simulink model "transfer_function_calculation"  (R2016a)
settings: Solver=VariableStepAuto  StartTime=0.0  StopTime=5  RelTol=1e-3
values from neighbouring files (symbols this model uses):
  a = .7    (= 0.7)    [PM_1_5MW_syn_27.m]
  Flux = 5.8264    [PM_1_5MW_syn_27.m]
  Id_set = 500    [PM_1_5MW_syn_27.m]
  Iq_set = -2200    [PM_1_5MW_syn_27.m]
  L = .0001    (= 0.0001)    [PM_1_5MW_syn_27.m]
  Ld = 0.001575    [PM_1_5MW_syn_27.m]
  Lq = 0.001575    [PM_1_5MW_syn_27.m]
  mn = 60000    [PM_1_5MW_syn_27.m]
  p = 26    [PM_1_5MW_syn_27.m]
  Rs = 0.000821    [PM_1_5MW_syn_27.m]
  Sollkurve_M_Optimum = [0 57121 101549 158670 228485 310994 406196 514092 634681 767965 810425 823386 ... (13 elements, 13x1)]    [Lookup_M_n.mat]
  Sollkurve_nGen_Optimum = [0 5 7 9 11 12 14 16 18 20 20.07 20.2 ... (13 elements, 13x1)]    [Lookup_M_n.mat]
  Speed_set = w_m    (= 2.10172548525)    [PM_1_5MW_syn_27.m]
  Ts_Power = 5.000000000000000e-06    (= 5e-06)    [PM_1_5MW_syn_27.m]
  Vdc = 1200    [PM_1_5MW_syn_27.m]
  Vh = Vm/6*0    (= 0)    [PM_1_5MW_syn_27.m]
undefined symbols (not defined in the file or in its folder): C2, Esw_Erec, Esw_Off, Esw_On, Page_Temp_C
undefined symbols (not defined in the file): Ts_Control, z
libraries: fl_lib x84, powerlib_meascontrol x58, simulink x56, nesl_utility x36, powerlib x33, simulink_extras x11
(part 4 of 6)

== system transfer_function_calculation/Generator/3 Level Converter2/Loss Calculation/Leg B1/Subsystem ==
  In1 : Inport
  In2 : Inport  Port=2
  Bus Creator : Subsystem
  Loss Calculation Unit : Subsystem
  Scope : Scope
  Scope1 : Scope
  Scope2 : Scope
  Conn1 : PMIOPort  Port=1  Side=Left
  Out1 : Outport
  wires:
  Loss Calculation Unit/3(Psw_IGBTs) -> Scope1/1, Bus Creator/3(In3)
  In1/1 -> Loss Calculation Unit/1(QD1)
  Loss Calculation Unit/1(mQd1) -> Bus Creator/1(In1)
  Loss Calculation Unit/9(Ptot_HB) -> Bus Creator/9(In9)
  Loss Calculation Unit/7(Pcond_diodes) -> Bus Creator/7(In7)
  Loss Calculation Unit/8(Ptot_Diodes) -> Bus Creator/8(In8)
  In2/1 -> Loss Calculation Unit/2(QD2)
  Loss Calculation Unit/11(TJ_Diodes) -> Bus Creator/11(In11)
  Loss Calculation Unit/10(TJ_IGBT) -> Bus Creator/10(In10)
  Loss Calculation Unit/6(Psw_Diodes) -> Scope2/1, Bus Creator/6(In6)
  Loss Calculation Unit/5(Ptot_IGBTs) -> Bus Creator/5(In5)
  Loss Calculation Unit/2(mQd2) -> Bus Creator/2(In2)
  Bus Creator/1(m) -> Out1/1
  Loss Calculation Unit/4(Pcond_IGBT) -> Bus Creator/4(In4), Scope/1
  Loss Calculation Unit/12(Tcase) -> Bus Creator/12(In12)
  connections:
  Conn1/RConn1 -- Loss Calculation Unit/RConn1

== system transfer_function_calculation/Generator/3 Level Converter2/Loss Calculation/Leg B2/Heat Sink (Simscape thermal model) ==
  Ta : Inport
  Conductive Heat Transfer Case 1 to Sink : fl_lib/Thermal/Thermal Elements/Conductive Heat Transfer  area=1 m^2  thickness=1 m  th_cond=1/Rth(1) W/(m*K)  Q_specify=off  Q_priority=High  Q=0 J/s  T_specify=off  T_priority=High  T=0 K
  Convective Heat Transfer Sink-to-Ambient : fl_lib/Thermal/Thermal Elements/Convective Heat Transfer  area=1 m^2  heat_tr_coeff=1/Rth(2) W/(m^2 * K)  Q_specify=off  Q_priority=High  Q=0 J/s  T_specify=off  T_priority=High  T=0 K
  PS2S : Subsystem
  PS2S1 : Subsystem
  S2PS1 : Subsystem
  Scope : Scope
  Scope1 : Scope
  Simscape Solver Configuration : nesl_utility/Solver Configuration  PhysicalDomain=network_engine_domain  SubClassName=solver  LeftPortType=input  RightPortType=generic  Accelerate=off  Tones=[]  Harmonics=[]  SimulateNoise=off  Profile=off  UseLocalSampling=off  EnableSwitchedLinearOptims=on  FrequencyDomain=off  UseCCode=off  RelTol=0.001  AbsTol=1e-06  MinStep=1e-09  ToWorkspace=off  RevertToSquareIcSolve=off  NumHomotopyIterations=100  PhasorMode=off  PhasorModeNumHarmonics=1  OverrideAbsTol=off  DoDC=off  ResidualTolerance=1e-9  UseLocalSolver=on  LocalSolverChoice=NE_TRAPEZOIDAL_ADVANCER  LocalSolverSampleTime=Ts_Control  DoFixedCost=off  MaxNonlinIter=2  MaxModeIter=1  LinearAlgebra=Sparse  DelaysMemoryBudget=1024  AutomaticFiltering=on  FilteringTimeConstant=0.001
  Temperature Sensor : fl_lib/Thermal/Thermal Sensors/Ideal Temperature Sensor
  Temperature Sensor1 : fl_lib/Thermal/Thermal Sensors/Ideal Temperature Sensor
  Temperature Source : fl_lib/Thermal/Thermal Sources/Ideal Temperature Source
  Thermal Reference : fl_lib/Thermal/Thermal Elements/Thermal Reference
  Thermal Reference1 : fl_lib/Thermal/Thermal Elements/Thermal Reference
  Thermal Reference2 : fl_lib/Thermal/Thermal Elements/Thermal Reference
  Thermal Mass (Case 1) : fl_lib/Thermal/Thermal Elements/Thermal Mass  mass=Cth(1) kg  sp_heat=1 J/kg/K  T_specify=on  T_priority=High  T=Tinit degC  Q_specify=off  Q_priority=High  Q=0 J/s
  Thermal Mass (Heatsink) : fl_lib/Thermal/Thermal Elements/Thermal Mass  mass=Cth(2) kg  sp_heat=1 J/kg/K  T_specify=on  T_priority=High  T=Tinit degC  Q_specify=off  Q_priority=High  Q=0 J/s
  H1 : PMIOPort  Port=1  Side=Right
  Tsink : Outport
  wires:
  PS2S1/1(Out) -> Scope1/1
  Ta/1 -> S2PS1/1(In), Scope/1
  PS2S/1(Out) -> Tsink/1
  connections:
  Temperature Sensor1/RConn2 -- PS2S1/LConn1
  Temperature Sensor1/RConn1 -- Thermal Reference2/LConn1
  H1/RConn1 -- Thermal Mass (Case 1)/LConn1 -- Conductive Heat Transfer Case 1 to Sink/LConn1
  Temperature Source/RConn2 -- Thermal Reference1/LConn1
  S2PS1/RConn1 -- Temperature Source/RConn1
  Temperature Source/LConn1 -- Temperature Sensor1/LConn1 -- Convective Heat Transfer Sink-to-Ambient/RConn1
  Temperature Sensor/LConn1 -- Convective Heat Transfer Sink-to-Ambient/LConn1 -- Thermal Mass (Heatsink)/LConn1 -- Conductive Heat Transfer Case 1 to Sink/RConn1 -- Simscape Solver Configuration/RConn1
  Temperature Sensor/RConn1 -- Thermal Reference/LConn1
  Temperature Sensor/RConn2 -- PS2S/LConn1

== system transfer_function_calculation/Generator/3 Level Converter2/Loss Calculation/Leg B2/Subsystem ==
  In1 : Inport
  In2 : Inport  Port=2
  Bus Creator : Subsystem
  Loss Calculation Unit : Subsystem
  Scope : Scope
  Scope1 : Scope
  Scope2 : Scope
  Conn1 : PMIOPort  Port=1  Side=Left
  Out1 : Outport
  wires:
  Loss Calculation Unit/12(Tcase) -> Bus Creator/12(In12)
  Loss Calculation Unit/4(Pcond_IGBT) -> Scope/1, Bus Creator/4(In4)
  Bus Creator/1(m) -> Out1/1
  Loss Calculation Unit/2(mQd2) -> Bus Creator/2(In2)
  Loss Calculation Unit/5(Ptot_IGBTs) -> Bus Creator/5(In5)
  Loss Calculation Unit/6(Psw_Diodes) -> Bus Creator/6(In6), Scope2/1
  Loss Calculation Unit/10(TJ_IGBT) -> Bus Creator/10(In10)
  Loss Calculation Unit/11(TJ_Diodes) -> Bus Creator/11(In11)
  In2/1 -> Loss Calculation Unit/2(QD2)
  Loss Calculation Unit/8(Ptot_Diodes) -> Bus Creator/8(In8)
  Loss Calculation Unit/7(Pcond_diodes) -> Bus Creator/7(In7)
  Loss Calculation Unit/9(Ptot_HB) -> Bus Creator/9(In9)
  Loss Calculation Unit/1(mQd1) -> Bus Creator/1(In1)
  In1/1 -> Loss Calculation Unit/1(QD1)
  Loss Calculation Unit/3(Psw_IGBTs) -> Bus Creator/3(In3), Scope1/1
  connections:
  Conn1/RConn1 -- Loss Calculation Unit/RConn1

== system transfer_function_calculation/Generator/3 Level Converter2/Loss Calculation/Leg C1/Heat Sink (Simscape thermal model) ==
  Ta : Inport
  Conductive Heat Transfer Case 1 to Sink : fl_lib/Thermal/Thermal Elements/Conductive Heat Transfer  area=1 m^2  thickness=1 m  th_cond=1/Rth(1) W/(m*K)  Q_specify=off  Q_priority=High  Q=0 J/s  T_specify=off  T_priority=High  T=0 K
  Convective Heat Transfer Sink-to-Ambient : fl_lib/Thermal/Thermal Elements/Convective Heat Transfer  area=1 m^2  heat_tr_coeff=1/Rth(2) W/(m^2 * K)  Q_specify=off  Q_priority=High  Q=0 J/s  T_specify=off  T_priority=High  T=0 K
  PS2S : Subsystem
  PS2S1 : Subsystem
  S2PS1 : Subsystem
  Scope : Scope
  Scope1 : Scope
  Simscape Solver Configuration : nesl_utility/Solver Configuration  PhysicalDomain=network_engine_domain  SubClassName=solver  LeftPortType=input  RightPortType=generic  Accelerate=off  Tones=[]  Harmonics=[]  SimulateNoise=off  Profile=off  UseLocalSampling=off  EnableSwitchedLinearOptims=on  FrequencyDomain=off  UseCCode=off  RelTol=0.001  AbsTol=1e-06  MinStep=1e-09  ToWorkspace=off  RevertToSquareIcSolve=off  NumHomotopyIterations=100  PhasorMode=off  PhasorModeNumHarmonics=1  OverrideAbsTol=off  DoDC=off  ResidualTolerance=1e-9  UseLocalSolver=on  LocalSolverChoice=NE_TRAPEZOIDAL_ADVANCER  LocalSolverSampleTime=Ts_Control  DoFixedCost=off  MaxNonlinIter=2  MaxModeIter=1  LinearAlgebra=Sparse  DelaysMemoryBudget=1024  AutomaticFiltering=on  FilteringTimeConstant=0.001
  Temperature Sensor : fl_lib/Thermal/Thermal Sensors/Ideal Temperature Sensor
  Temperature Sensor1 : fl_lib/Thermal/Thermal Sensors/Ideal Temperature Sensor
  Temperature Source : fl_lib/Thermal/Thermal Sources/Ideal Temperature Source
  Thermal Reference : fl_lib/Thermal/Thermal Elements/Thermal Reference
  Thermal Reference1 : fl_lib/Thermal/Thermal Elements/Thermal Reference
  Thermal Reference2 : fl_lib/Thermal/Thermal Elements/Thermal Reference
  Thermal Mass (Case 1) : fl_lib/Thermal/Thermal Elements/Thermal Mass  mass=Cth(1) kg  sp_heat=1 J/kg/K  T_specify=on  T_priority=High  T=Tinit degC  Q_specify=off  Q_priority=High  Q=0 J/s
  Thermal Mass (Heatsink) : fl_lib/Thermal/Thermal Elements/Thermal Mass  mass=Cth(2) kg  sp_heat=1 J/kg/K  T_specify=on  T_priority=High  T=Tinit degC  Q_specify=off  Q_priority=High  Q=0 J/s
  H1 : PMIOPort  Port=1  Side=Right
  Tsink : Outport
  wires:
  PS2S/1(Out) -> Tsink/1
  Ta/1 -> Scope/1, S2PS1/1(In)
  PS2S1/1(Out) -> Scope1/1
  connections:
  Temperature Sensor/RConn2 -- PS2S/LConn1
  Temperature Sensor/RConn1 -- Thermal Reference/LConn1
  Simscape Solver Configuration/RConn1 -- Conductive Heat Transfer Case 1 to Sink/RConn1 -- Thermal Mass (Heatsink)/LConn1 -- Convective Heat Transfer Sink-to-Ambient/LConn1 -- Temperature Sensor/LConn1
  Convective Heat Transfer Sink-to-Ambient/RConn1 -- Temperature Sensor1/LConn1 -- Temperature Source/LConn1
  S2PS1/RConn1 -- Temperature Source/RConn1
  Temperature Source/RConn2 -- Thermal Reference1/LConn1
  Conductive Heat Transfer Case 1 to Sink/LConn1 -- Thermal Mass (Case 1)/LConn1 -- H1/RConn1
  Temperature Sensor1/RConn1 -- Thermal Reference2/LConn1
  Temperature Sensor1/RConn2 -- PS2S1/LConn1

== system transfer_function_calculation/Generator/3 Level Converter2/Loss Calculation/Leg C1/Subsystem ==
  In1 : Inport
  In2 : Inport  Port=2
  Bus Creator : Subsystem
  Loss Calculation Unit : Subsystem
  Scope : Scope
  Scope1 : Scope
  Scope2 : Scope
  Conn1 : PMIOPort  Port=1  Side=Left
  Out1 : Outport
  wires:
  Loss Calculation Unit/3(Psw_IGBTs) -> Scope1/1, Bus Creator/3(In3)
  In1/1 -> Loss Calculation Unit/1(QD1)
  Loss Calculation Unit/1(mQd1) -> Bus Creator/1(In1)
  Loss Calculation Unit/9(Ptot_HB) -> Bus Creator/9(In9)
  Loss Calculation Unit/7(Pcond_diodes) -> Bus Creator/7(In7)
  Loss Calculation Unit/8(Ptot_Diodes) -> Bus Creator/8(In8)
  In2/1 -> Loss Calculation Unit/2(QD2)
  Loss Calculation Unit/11(TJ_Diodes) -> Bus Creator/11(In11)
  Loss Calculation Unit/10(TJ_IGBT) -> Bus Creator/10(In10)
  Loss Calculation Unit/6(Psw_Diodes) -> Scope2/1, Bus Creator/6(In6)
  Loss Calculation Unit/5(Ptot_IGBTs) -> Bus Creator/5(In5)
  Loss Calculation Unit/2(mQd2) -> Bus Creator/2(In2)
  Bus Creator/1(m) -> Out1/1
  Loss Calculation Unit/4(Pcond_IGBT) -> Bus Creator/4(In4), Scope/1
  Loss Calculation Unit/12(Tcase) -> Bus Creator/12(In12)
  connections:
  Conn1/RConn1 -- Loss Calculation Unit/RConn1

== system transfer_function_calculation/Generator/3 Level Converter2/Loss Calculation/Leg C2/Heat Sink (Simscape thermal model) ==
  Ta : Inport
  Conductive Heat Transfer Case 1 to Sink : fl_lib/Thermal/Thermal Elements/Conductive Heat Transfer  area=1 m^2  thickness=1 m  th_cond=1/Rth(1) W/(m*K)  Q_specify=off  Q_priority=High  Q=0 J/s  T_specify=off  T_priority=High  T=0 K
  Convective Heat Transfer Sink-to-Ambient : fl_lib/Thermal/Thermal Elements/Convective Heat Transfer  area=1 m^2  heat_tr_coeff=1/Rth(2) W/(m^2 * K)  Q_specify=off  Q_priority=High  Q=0 J/s  T_specify=off  T_priority=High  T=0 K
  PS2S : Subsystem
  PS2S1 : Subsystem
  S2PS1 : Subsystem
  Scope : Scope
  Scope1 : Scope
  Simscape Solver Configuration : nesl_utility/Solver Configuration  PhysicalDomain=network_engine_domain  SubClassName=solver  LeftPortType=input  RightPortType=generic  Accelerate=off  Tones=[]  Harmonics=[]  SimulateNoise=off  Profile=off  UseLocalSampling=off  EnableSwitchedLinearOptims=on  FrequencyDomain=off  UseCCode=off  RelTol=0.001  AbsTol=1e-06  MinStep=1e-09  ToWorkspace=off  RevertToSquareIcSolve=off  NumHomotopyIterations=100  PhasorMode=off  PhasorModeNumHarmonics=1  OverrideAbsTol=off  DoDC=off  ResidualTolerance=1e-9  UseLocalSolver=on  LocalSolverChoice=NE_TRAPEZOIDAL_ADVANCER  LocalSolverSampleTime=Ts_Control  DoFixedCost=off  MaxNonlinIter=2  MaxModeIter=1  LinearAlgebra=Sparse  DelaysMemoryBudget=1024  AutomaticFiltering=on  FilteringTimeConstant=0.001
  Temperature Sensor : fl_lib/Thermal/Thermal Sensors/Ideal Temperature Sensor
  Temperature Sensor1 : fl_lib/Thermal/Thermal Sensors/Ideal Temperature Sensor
  Temperature Source : fl_lib/Thermal/Thermal Sources/Ideal Temperature Source
  Thermal Reference : fl_lib/Thermal/Thermal Elements/Thermal Reference
  Thermal Reference1 : fl_lib/Thermal/Thermal Elements/Thermal Reference
  Thermal Reference2 : fl_lib/Thermal/Thermal Elements/Thermal Reference
  Thermal Mass (Case 1) : fl_lib/Thermal/Thermal Elements/Thermal Mass  mass=Cth(1) kg  sp_heat=1 J/kg/K  T_specify=on  T_priority=High  T=Tinit degC  Q_specify=off  Q_priority=High  Q=0 J/s
  Thermal Mass (Heatsink) : fl_lib/Thermal/Thermal Elements/Thermal Mass  mass=Cth(2) kg  sp_heat=1 J/kg/K  T_specify=on  T_priority=High  T=Tinit degC  Q_specify=off  Q_priority=High  Q=0 J/s
  H1 : PMIOPort  Port=1  Side=Right
  Tsink : Outport
  wires:
  PS2S1/1(Out) -> Scope1/1
  Ta/1 -> S2PS1/1(In), Scope/1
  PS2S/1(Out) -> Tsink/1
  connections:
  Temperature Sensor1/RConn2 -- PS2S1/LConn1
  Temperature Sensor1/RConn1 -- Thermal Reference2/LConn1
  H1/RConn1 -- Thermal Mass (Case 1)/LConn1 -- Conductive Heat Transfer Case 1 to Sink/LConn1
  Temperature Source/RConn2 -- Thermal Reference1/LConn1
  S2PS1/RConn1 -- Temperature Source/RConn1
  Temperature Source/LConn1 -- Temperature Sensor1/LConn1 -- Convective Heat Transfer Sink-to-Ambient/RConn1
  Temperature Sensor/LConn1 -- Convective Heat Transfer Sink-to-Ambient/LConn1 -- Thermal Mass (Heatsink)/LConn1 -- Conductive Heat Transfer Case 1 to Sink/RConn1 -- Simscape Solver Configuration/RConn1
  Temperature Sensor/RConn1 -- Thermal Reference/LConn1
  Temperature Sensor/RConn2 -- PS2S/LConn1

== system transfer_function_calculation/Generator/3 Level Converter2/Loss Calculation/Leg C2/Subsystem ==
  In1 : Inport
  In2 : Inport  Port=2
  Bus Creator : Subsystem
  Loss Calculation Unit : Subsystem
  Scope : Scope
  Scope1 : Scope
  Scope2 : Scope
  Conn1 : PMIOPort  Port=1  Side=Left
  Out1 : Outport
  wires:
  Loss Calculation Unit/12(Tcase) -> Bus Creator/12(In12)
  Loss Calculation Unit/4(Pcond_IGBT) -> Scope/1, Bus Creator/4(In4)
  Bus Creator/1(m) -> Out1/1
  Loss Calculation Unit/2(mQd2) -> Bus Creator/2(In2)
  Loss Calculation Unit/5(Ptot_IGBTs) -> Bus Creator/5(In5)
  Loss Calculation Unit/6(Psw_Diodes) -> Bus Creator/6(In6), Scope2/1
  Loss Calculation Unit/10(TJ_IGBT) -> Bus Creator/10(In10)
  Loss Calculation Unit/11(TJ_Diodes) -> Bus Creator/11(In11)
  In2/1 -> Loss Calculation Unit/2(QD2)
  Loss Calculation Unit/8(Ptot_Diodes) -> Bus Creator/8(In8)
  Loss Calculation Unit/7(Pcond_diodes) -> Bus Creator/7(In7)
  Loss Calculation Unit/9(Ptot_HB) -> Bus Creator/9(In9)
  Loss Calculation Unit/1(mQd1) -> Bus Creator/1(In1)
  In1/1 -> Loss Calculation Unit/1(QD1)
  Loss Calculation Unit/3(Psw_IGBTs) -> Bus Creator/3(In3), Scope1/1
  connections:
  Conn1/RConn1 -- Loss Calculation Unit/RConn1

== system transfer_function_calculation/Generator/3 Level Converter2/Loss Calculation/Leg A1/Heat Sink (Simscape thermal model)/PS2S ==
  Add1 : Sum  Inputs=+-
  K1 : Constant  Value=273
  PS-Simulink Converter : nesl_utility/PS-Simulink Converter  PhysicalDomain=network_engine_domain  SubClassName=ps_output  LeftPortType=input  RightPortType=output  PseudoPeriodic=off  Frequencies=[]  Unit=1  AffineConversion=off
  In : PMIOPort  Port=1  Side=Left
  Out : Outport
  wires:
  K1/1 -> Add1/2
  PS-Simulink Converter/1 -> Add1/1
  Add1/1 -> Out/1
  connections:
  In/RConn1 -- PS-Simulink Converter/LConn1

== system transfer_function_calculation/Generator/3 Level Converter2/Loss Calculation/Leg A1/Heat Sink (Simscape thermal model)/PS2S1 ==
  Add1 : Sum  Inputs=+-
  K1 : Constant  Value=273
  PS-Simulink Converter : nesl_utility/PS-Simulink Converter  PhysicalDomain=network_engine_domain  SubClassName=ps_output  LeftPortType=input  RightPortType=output  PseudoPeriodic=off  Frequencies=[]  Unit=1  AffineConversion=off
  In : PMIOPort  Port=1  Side=Left
  Out : Outport
  wires:
  Add1/1 -> Out/1
  PS-Simulink Converter/1 -> Add1/1
  K1/1 -> Add1/2
  connections:
  In/RConn1 -- PS-Simulink Converter/LConn1

== system transfer_function_calculation/Generator/3 Level Converter2/Loss Calculation/Leg A1/Heat Sink (Simscape thermal model)/S2PS1 ==
  In : Inport
  Add : Sum
  K2 : Constant  Value=273
  Simulink-PS Converter : nesl_utility/Simulink-PS Converter  PhysicalDomain=network_engine_domain  SubClassName=ps_input  LeftPortType=input  RightPortType=output  PseudoPeriodic=off  Frequencies=[]  NoiseDistribution=none  NoiseParameters=[]  Unit=1  AffineConversion=off  InputFiltering=off  SimscapeFilterOrder=1  InputFilterTimeConstant=1e-4  UdotUserProvided=0
  Out : PMIOPort  Port=1  Side=Right
  wires:
  Add/1 -> Simulink-PS Converter/1
  K2/1 -> Add/1
  In/1 -> Add/2
  connections:
  Out/RConn1 -- Simulink-PS Converter/RConn1

== system transfer_function_calculation/Generator/3 Level Converter2/Loss Calculation/Leg A1/Subsystem/Bus Creator ==
  In1 : Inport
  In2 : Inport  Port=2
  In3 : Inport  Port=3
  In4 : Inport  Port=4
  In5 : Inport  Port=5
  In6 : Inport  Port=6
  In7 : Inport  Port=7
  In8 : Inport  Port=8
  In9 : Inport  Port=9
  In10 : Inport  Port=10
  In11 : Inport  Port=11
  In12 : Inport  Port=12
  Bus Creator : BusCreator  Inputs=22
  Demux{1..10} (10 alike) : Demux  Outputs=2
  Scope : Scope  NumInputPorts=4
  m : Outport
  wires:
  Demux4/2 -> Bus Creator/12  "Psw_Diode2"
  Demux2/2 -> Bus Creator/6  "Psw_IGBT2"
  Demux8/1 -> Bus Creator/20  "Tj_Diode1"
  In2/1 -> Demux9/1
  Demux9/2 -> Bus Creator/4  "V_Dev2"
  In1/1 -> Demux10/1
  Demux1/1 -> Bus Creator/7  "Pcond_IGBT1"
  Demux5/1 -> Bus Creator/13  "Pcond_Diode1"
  Demux2/1 -> Bus Creator/5  "Psw_IGBT1"
  Demux7/2 -> Bus Creator/19  "Tj_IGBT2"
  In11/1 -> Demux8/1
  Demux9/1 -> Bus Creator/3  "I_Dev2"
  In4/1 -> Demux1/1
  In7/1 -> Demux5/1
  Demux10/1 -> Bus Creator/1  "I_Dev1"
  In3/1 -> Demux2/1
  Demux7/1 -> Bus Creator/18  "Tj_IGBT1"
  In9/1 -> Bus Creator/17  "Ptot_HalfBridge"
  In10/1 -> Demux7/1
  Demux4/1 -> Bus Creator/11  "Psw_Diode1"
  In12/1 -> Bus Creator/22  "Tcase"
  Demux6/1 -> Scope/2, [D1], Bus Creator/15  "Ptot_Diode1"
  In8/1 -> Demux6/1
  Demux6/2 -> Scope/1, [D2], Bus Creator/16  "Ptot_Diode2"
  Demux3/2 -> Scope/3, [IGBT2], Bus Creator/10  "Ptot_IGBT2"
  Demux10/2 -> Bus Creator/2  "V_Dev1"
  Demux1/2 -> Bus Creator/8  "Pcond_IGBT2"
  In5/1 -> Demux3/1
  Demux3/1 -> Scope/4, [IGBT1], Bus Creator/9  "Ptot_IGBT1"
  Demux5/2 -> Bus Creator/14  "Pcond_Diode2"
  Bus Creator/1 -> m/1
  Demux8/2 -> Bus Creator/21  "Tj_Diode2"
  In6/1 -> Demux4/1

== system transfer_function_calculation/Generator/3 Level Converter2/Loss Calculation/Leg A1/Subsystem/Loss Calculation Unit ==
  From m point of  IGBT1 : Inport
  From m point of  IGBT2 : Inport  Port=2
  Add1 : Sum
  Add2 : Sum  Inputs=+
  Add3 : Sum  Inputs=+-
  Add4 : Sum  Inputs=+
  Demux IGBTs and Diodes Currents and voltages : Subsystem
  Diodes Losses Calculation : Subsystem
  Heat Flow Source : fl_lib/Thermal/Thermal Sources/Ideal Heat Flow Source
  IGBTs Losses Calculation : Subsystem
  K1 : Constant  Value=273
  PS-Simulink Converter : nesl_utility/PS-Simulink Converter  PhysicalDomain=network_engine_domain  SubClassName=ps_output  LeftPortType=input  RightPortType=output  PseudoPeriodic=off  Frequencies=[]  Unit=1  AffineConversion=off
  Rate Transition : RateTransition  OutPortSampleTime=Ts_Simscape
  Rate Transition1 : RateTransition  OutPortSampleTime=Ts
  Simulink-PS Converter1 : nesl_utility/Simulink-PS Converter  PhysicalDomain=network_engine_domain  SubClassName=ps_input  LeftPortType=input  RightPortType=output  PseudoPeriodic=off  Frequencies=[]  NoiseDistribution=none  NoiseParameters=[]  Unit=1  AffineConversion=off  InputFiltering=off  SimscapeFilterOrder=1  InputFilterTimeConstant=1e-4  UdotUserProvided=0
  Temperature Sensor : fl_lib/Thermal/Thermal Sensors/Ideal Temperature Sensor
  Thermal Reference1 : fl_lib/Thermal/Thermal Elements/Thermal Reference
  Thermal Reference4 : fl_lib/Thermal/Thermal Elements/Thermal Reference
  Thermal Model : Subsystem  mask(State-Space Thermal Model (Junction-to-Case)){Zth_IGBT=[ IGBT_Rth_jc    IGBT_Cth_j ], Zth_Diode=[ DIODE_Rth_jc    DIODE_Cth_j], Tj0=Tj0, Ts=Ts}
      mask prompts: Zth_IGBT "IGBT Thermal Impedance [ Rth (K/W)  Cth (J/K) ]:"; Zth_Diode "Diode Thermal Impedance [ Rth (K/W)  Cth (J/K) ]:"; Tj0 "Junction Initial Temperature (C)"; Ts "Sample time (s):"
      mask init:
      | %
      | Rth_IGBT= Zth_IGBT(1);
      | Cth_IGBT= Zth_IGBT(2);
      | Rth_Diode= Zth_Diode(1);
      | Cth_Diode= Zth_Diode(2);
      | %
      | Ac_IGBT= -1/(Rth_IGBT*Cth_IGBT);
      | Bc_IGBT= [ 1/(Rth_IGBT*Cth_IGBT)  1/Cth_IGBT ];
      | Cc_IGBT= [ 1; 1/Rth_IGBT ];
      | Dc_IGBT= [ 0  0; -1/Rth_IGBT 0 ];
      | %
      | Ac_Diode= -1/(Rth_Diode*Cth_Diode);
      | Bc_Diode= [ 1/(Rth_Diode*Cth_Diode)  1/Cth_Diode ];
      | Cc_Diode= [ 1; 1/Rth_Diode ];
      | Dc_Diode= [ 0  0; -1/Rth_Diode 0 ];
      | %
      | x0c=Tj0;
      | %
      | %  Conversion to discrete transfer function
      | nstates = size(Ac_IGBT,1);
      | invexp = inv(eye(nstates) - (Ts/2)*Ac_IGBT);
      | Ad_IGBT = invexp*(eye(nstates) + (Ts/2)*Ac_IGBT);
      | Bd_IGBT = invexp*Bc_IGBT;
      | Cd_IGBT = Cc_IGBT*invexp*Ts;
      | Dd_IGBT = Cc_IGBT*invexp*Bc_IGBT*(Ts/2) + Dc_IGBT;
      | %
      | x0c=Tj0;
      | I=eye(size(Ac_IGBT));
      | x0d=(I-Ac_IGBT*Ts/2)*x0c/Ts;
      | %
      | %  Conversion to discrete transfer function
      | nstates = size(Ac_Diode,1);
      | invexp = inv(eye(nstates) - (Ts/2)*Ac_Diode);
      | Ad_Diode = invexp*(eye(nstates) + (Ts/2)*Ac_Diode);
      | Bd_Diode = invexp*Bc_Diode;
      | Cd_Diode = Cc_Diode*invexp*Ts;
      | Dd_Diode = Cc_Diode*invexp*Bc_Diode*(Ts/2) + Dc_Diode;
      | %
  HA1 : PMIOPort  Port=1  Side=Right
  mQd1 : Outport
  mQd2 : Outport  Port=2
  Psw_IGBTs : Outport  Port=3
  Pcond_IGBT : Outport  Port=4
  Ptot_IGBTs : Outport  Port=5
  Psw_Diodes : Outport  Port=6
  Pcond_diodes : Outport  Port=7
  Ptot_Diodes : Outport  Port=8
  Ptot_HB : Outport  Port=9
  TJ_IGBT : Outport  Port=10
  TJ_Diodes : Outport  Port=11
  Tcase : Outport  Port=12
  wires:
  Rate Transition/1 -> Simulink-PS Converter1/1
  Thermal Model/2(Pout) -> Rate Transition/1
  K1/1 -> Add3/2
  PS-Simulink Converter/1 -> Add3/1
  Add3/1 -> Rate Transition1/1, Tcase/1
  Thermal Model/1(Tj_IGBTs) -> IGBTs Losses Calculation/1(Tj_C), TJ_IGBT/1
  Thermal Model/3(Tj_Diodes) -> Diodes Losses Calculation/2(Tj_C), TJ_Diodes/1
  IGBTs Losses Calculation/1(Psw) -> Psw_IGBTs/1
  Diodes Losses Calculation/2(Psw) -> Psw_Diodes/1
  Diodes Losses Calculation/3(Pcond) -> Pcond_diodes/1
  Add1/1 -> Ptot_HB/1
  Add4/1 -> Add1/1
  Add2/1 -> Add1/2
  Rate Transition1/1 -> Thermal Model/3(Tcase)
  Demux IGBTs and Diodes Currents and voltages/2(Diodes) -> Diodes Losses Calculation/1(i,v)
  Demux IGBTs and Diodes Currents and voltages/1(IGBTs) -> IGBTs Losses Calculation/2(i,v)
  From m point of  IGBT2/1 -> Demux IGBTs and Diodes Currents and voltages/2(QD2), mQd2/1
  From m point of  IGBT1/1 -> mQd1/1, Demux IGBTs and Diodes Currents and voltages/1(QD1)
  IGBTs Losses Calculation/2(Pcond) -> Pcond_IGBT/1
  Diodes Losses Calculation/1(Ptot) -> Add2/1, Thermal Model/2(P_Diodes), Ptot_Diodes/1
  IGBTs Losses Calculation/3(Ptot) -> Add4/1, Thermal Model/1(P_IGBTs), Ptot_IGBTs/1
  connections:
  Temperature Sensor/RConn1 -- Thermal Reference1/LConn1
  Temperature Sensor/RConn2 -- PS-Simulink Converter/LConn1
  Simulink-PS Converter1/RConn1 -- Heat Flow Source/RConn1
  Thermal Reference4/LConn1 -- Heat Flow Source/RConn2
  Temperature Sensor/LConn1 -- HA1/RConn1 -- Heat Flow Source/LConn1

== system transfer_function_calculation/Generator/3 Level Converter2/Loss Calculation/Leg A2/Heat Sink (Simscape thermal model)/PS2S ==
  Add1 : Sum  Inputs=+-
  K1 : Constant  Value=273
  PS-Simulink Converter : nesl_utility/PS-Simulink Converter  PhysicalDomain=network_engine_domain  SubClassName=ps_output  LeftPortType=input  RightPortType=output  PseudoPeriodic=off  Frequencies=[]  Unit=1  AffineConversion=off
  In : PMIOPort  Port=1  Side=Left
  Out : Outport
  wires:
  Add1/1 -> Out/1
  PS-Simulink Converter/1 -> Add1/1
  K1/1 -> Add1/2
  connections:
  In/RConn1 -- PS-Simulink Converter/LConn1

== system transfer_function_calculation/Generator/3 Level Converter2/Loss Calculation/Leg A2/Heat Sink (Simscape thermal model)/PS2S1 ==
  Add1 : Sum  Inputs=+-
  K1 : Constant  Value=273
  PS-Simulink Converter : nesl_utility/PS-Simulink Converter  PhysicalDomain=network_engine_domain  SubClassName=ps_output  LeftPortType=input  RightPortType=output  PseudoPeriodic=off  Frequencies=[]  Unit=1  AffineConversion=off
  In : PMIOPort  Port=1  Side=Left
  Out : Outport
  wires:
  K1/1 -> Add1/2
  PS-Simulink Converter/1 -> Add1/1
  Add1/1 -> Out/1
  connections:
  In/RConn1 -- PS-Simulink Converter/LConn1

== system transfer_function_calculation/Generator/3 Level Converter2/Loss Calculation/Leg A2/Heat Sink (Simscape thermal model)/S2PS1 ==
  In : Inport
  Add : Sum
  K2 : Constant  Value=273
  Simulink-PS Converter : nesl_utility/Simulink-PS Converter  PhysicalDomain=network_engine_domain  SubClassName=ps_input  LeftPortType=input  RightPortType=output  PseudoPeriodic=off  Frequencies=[]  NoiseDistribution=none  NoiseParameters=[]  Unit=1  AffineConversion=off  InputFiltering=off  SimscapeFilterOrder=1  InputFilterTimeConstant=1e-4  UdotUserProvided=0
  Out : PMIOPort  Port=1  Side=Right
  wires:
  In/1 -> Add/2
  K2/1 -> Add/1
  Add/1 -> Simulink-PS Converter/1
  connections:
  Out/RConn1 -- Simulink-PS Converter/RConn1

== system transfer_function_calculation/Generator/3 Level Converter2/Loss Calculation/Leg A2/Subsystem/Bus Creator ==
  In1 : Inport
  In2 : Inport  Port=2
  In3 : Inport  Port=3
  In4 : Inport  Port=4
  In5 : Inport  Port=5
  In6 : Inport  Port=6
  In7 : Inport  Port=7
  In8 : Inport  Port=8
  In9 : Inport  Port=9
  In10 : Inport  Port=10
  In11 : Inport  Port=11
  In12 : Inport  Port=12
  Bus Creator : BusCreator  Inputs=22
  Demux{1..10} (10 alike) : Demux  Outputs=2
  Scope : Scope  NumInputPorts=4
  m : Outport
  wires:
  In6/1 -> Demux4/1
  Demux8/2 -> Bus Creator/21  "Tj_Diode2"
  Bus Creator/1 -> m/1
  Demux5/2 -> Bus Creator/14  "Pcond_Diode2"
  Demux3/1 -> Bus Creator/9, [IGBT1], Scope/4  "Ptot_IGBT1"
  In5/1 -> Demux3/1
  Demux1/2 -> Bus Creator/8  "Pcond_IGBT2"
  Demux10/2 -> Bus Creator/2  "V_Dev1"
  Demux3/2 -> Bus Creator/10, [IGBT2], Scope/3  "Ptot_IGBT2"
  Demux6/2 -> Bus Creator/16, [D2], Scope/1  "Ptot_Diode2"
  In8/1 -> Demux6/1
  Demux6/1 -> Bus Creator/15, [D1], Scope/2  "Ptot_Diode1"
  In12/1 -> Bus Creator/22  "Tcase"
  Demux4/1 -> Bus Creator/11  "Psw_Diode1"
  In10/1 -> Demux7/1
  In9/1 -> Bus Creator/17  "Ptot_HalfBridge"
  Demux7/1 -> Bus Creator/18  "Tj_IGBT1"
  In3/1 -> Demux2/1
  Demux10/1 -> Bus Creator/1  "I_Dev1"
  In7/1 -> Demux5/1
  In4/1 -> Demux1/1
  Demux9/1 -> Bus Creator/3  "I_Dev2"
  In11/1 -> Demux8/1
  Demux7/2 -> Bus Creator/19  "Tj_IGBT2"
  Demux2/1 -> Bus Creator/5  "Psw_IGBT1"
  Demux5/1 -> Bus Creator/13  "Pcond_Diode1"
  Demux1/1 -> Bus Creator/7  "Pcond_IGBT1"
  In1/1 -> Demux10/1
  Demux9/2 -> Bus Creator/4  "V_Dev2"
  In2/1 -> Demux9/1
  Demux8/1 -> Bus Creator/20  "Tj_Diode1"
  Demux2/2 -> Bus Creator/6  "Psw_IGBT2"
  Demux4/2 -> Bus Creator/12  "Psw_Diode2"

== system transfer_function_calculation/Generator/3 Level Converter2/Loss Calculation/Leg A2/Subsystem/Loss Calculation Unit ==
  QD1 : Inport
  QD2 : Inport  Port=2
  Add1 : Sum
  Add2 : Sum  Inputs=+
  Add3 : Sum  Inputs=+-
  Add4 : Sum  Inputs=+
  Demux IGBTs and Diodes Currents and voltages : Subsystem
  Diodes Losses Calculation : Subsystem
  Heat Flow Source : fl_lib/Thermal/Thermal Sources/Ideal Heat Flow Source
  IGBTs Losses Calculation : Subsystem
  K1 : Constant  Value=273
  PS-Simulink Converter : nesl_utility/PS-Simulink Converter  PhysicalDomain=network_engine_domain  SubClassName=ps_output  LeftPortType=input  RightPortType=output  PseudoPeriodic=off  Frequencies=[]  Unit=1  AffineConversion=off
  Rate Transition : RateTransition  OutPortSampleTime=Ts_Simscape
  Rate Transition1 : RateTransition  OutPortSampleTime=Ts
  Simulink-PS Converter1 : nesl_utility/Simulink-PS Converter  PhysicalDomain=network_engine_domain  SubClassName=ps_input  LeftPortType=input  RightPortType=output  PseudoPeriodic=off  Frequencies=[]  NoiseDistribution=none  NoiseParameters=[]  Unit=1  AffineConversion=off  InputFiltering=off  SimscapeFilterOrder=1  InputFilterTimeConstant=1e-4  UdotUserProvided=0
  Temperature Sensor : fl_lib/Thermal/Thermal Sensors/Ideal Temperature Sensor
  Thermal Reference1 : fl_lib/Thermal/Thermal Elements/Thermal Reference
  Thermal Reference4 : fl_lib/Thermal/Thermal Elements/Thermal Reference
  Thermal Model : Subsystem  mask(State-Space Thermal Model (Junction-to-Case)){Zth_IGBT=[ IGBT_Rth_jc    IGBT_Cth_j ], Zth_Diode=[ DIODE_Rth_jc    DIODE_Cth_j], Tj0=Tj0, Ts=Ts}
      mask prompts: Zth_IGBT "IGBT Thermal Impedance [ Rth (K/W)  Cth (J/K) ]:"; Zth_Diode "Diode Thermal Impedance [ Rth (K/W)  Cth (J/K) ]:"; Tj0 "Junction Initial Temperature (C)"; Ts "Sample time (s):"
      mask init: same as transfer_function_calculation/Generator/3 Level Converter2/Loss Calculation/Leg A1/Subsystem/Loss Calculation Unit/Thermal Model
  HA1 : PMIOPort  Port=1  Side=Right
  mQd1 : Outport
  mQd2 : Outport  Port=2
  Psw_IGBTs : Outport  Port=3
  Pcond_IGBT : Outport  Port=4
  Ptot_IGBTs : Outport  Port=5
  Psw_Diodes : Outport  Port=6
  Pcond_diodes : Outport  Port=7
  Ptot_Diodes : Outport  Port=8
  Ptot_HB : Outport  Port=9
  TJ_IGBT : Outport  Port=10
  TJ_Diodes : Outport  Port=11
  Tcase : Outport  Port=12
  wires:
  IGBTs Losses Calculation/3(Ptot) -> Ptot_IGBTs/1, Thermal Model/1(P_IGBTs), Add4/1
  Diodes Losses Calculation/1(Ptot) -> Ptot_Diodes/1, Thermal Model/2(P_Diodes), Add2/1
  IGBTs Losses Calculation/2(Pcond) -> Pcond_IGBT/1
  QD1/1 -> mQd1/1, Demux IGBTs and Diodes Currents and voltages/1(QD1)
  QD2/1 -> mQd2/1, Demux IGBTs and Diodes Currents and voltages/2(QD2)
  Demux IGBTs and Diodes Currents and voltages/1(IGBTs) -> IGBTs Losses Calculation/2(i,v)
  Demux IGBTs and Diodes Currents and voltages/2(Diodes) -> Diodes Losses Calculation/1(i,v)
  Rate Transition1/1 -> Thermal Model/3(Tcase)
  Add2/1 -> Add1/2
  Add4/1 -> Add1/1
  Add1/1 -> Ptot_HB/1
  Diodes Losses Calculation/3(Pcond) -> Pcond_diodes/1
  Diodes Losses Calculation/2(Psw) -> Psw_Diodes/1
  IGBTs Losses Calculation/1(Psw) -> Psw_IGBTs/1
  Thermal Model/3(Tj_Diodes) -> TJ_Diodes/1, Diodes Losses Calculation/2(Tj_C)
  Thermal Model/1(Tj_IGBTs) -> TJ_IGBT/1, IGBTs Losses Calculation/1(Tj_C)
  Add3/1 -> Tcase/1, Rate Transition1/1
  PS-Simulink Converter/1 -> Add3/1
  K1/1 -> Add3/2
  Thermal Model/2(Pout) -> Rate Transition/1
  Rate Transition/1 -> Simulink-PS Converter1/1
  connections:
  Heat Flow Source/LConn1 -- HA1/RConn1 -- Temperature Sensor/LConn1
  Thermal Reference4/LConn1 -- Heat Flow Source/RConn2
  Simulink-PS Converter1/RConn1 -- Heat Flow Source/RConn1
  Temperature Sensor/RConn2 -- PS-Simulink Converter/LConn1
  Temperature Sensor/RConn1 -- Thermal Reference1/LConn1

== system transfer_function_calculation/Generator/3 Level Converter2/Loss Calculation/Leg B1/Heat Sink (Simscape thermal model)/PS2S ==
  Add1 : Sum  Inputs=+-
  K1 : Constant  Value=273
  PS-Simulink Converter : nesl_utility/PS-Simulink Converter  PhysicalDomain=network_engine_domain  SubClassName=ps_output  LeftPortType=input  RightPortType=output  PseudoPeriodic=off  Frequencies=[]  Unit=1  AffineConversion=off
  In : PMIOPort  Port=1  Side=Left
  Out : Outport
  wires:
  K1/1 -> Add1/2
  PS-Simulink Converter/1 -> Add1/1
  Add1/1 -> Out/1
  connections:
  In/RConn1 -- PS-Simulink Converter/LConn1

== system transfer_function_calculation/Generator/3 Level Converter2/Loss Calculation/Leg B1/Heat Sink (Simscape thermal model)/PS2S1 ==
  Add1 : Sum  Inputs=+-
  K1 : Constant  Value=273
  PS-Simulink Converter : nesl_utility/PS-Simulink Converter  PhysicalDomain=network_engine_domain  SubClassName=ps_output  LeftPortType=input  RightPortType=output  PseudoPeriodic=off  Frequencies=[]  Unit=1  AffineConversion=off
  In : PMIOPort  Port=1  Side=Left
  Out : Outport
  wires:
  Add1/1 -> Out/1
  PS-Simulink Converter/1 -> Add1/1
  K1/1 -> Add1/2
  connections:
  In/RConn1 -- PS-Simulink Converter/LConn1

== system transfer_function_calculation/Generator/3 Level Converter2/Loss Calculation/Leg B1/Heat Sink (Simscape thermal model)/S2PS1 ==
  In : Inport
  Add : Sum
  K2 : Constant  Value=273
  Simulink-PS Converter : nesl_utility/Simulink-PS Converter  PhysicalDomain=network_engine_domain  SubClassName=ps_input  LeftPortType=input  RightPortType=output  PseudoPeriodic=off  Frequencies=[]  NoiseDistribution=none  NoiseParameters=[]  Unit=1  AffineConversion=off  InputFiltering=off  SimscapeFilterOrder=1  InputFilterTimeConstant=1e-4  UdotUserProvided=0
  Out : PMIOPort  Port=1  Side=Right
  wires:
  Add/1 -> Simulink-PS Converter/1
  K2/1 -> Add/1
  In/1 -> Add/2
  connections:
  Out/RConn1 -- Simulink-PS Converter/RConn1

== system transfer_function_calculation/Generator/3 Level Converter2/Loss Calculation/Leg B1/Subsystem/Bus Creator ==
  In1 : Inport
  In2 : Inport  Port=2
  In3 : Inport  Port=3
  In4 : Inport  Port=4
  In5 : Inport  Port=5
  In6 : Inport  Port=6
  In7 : Inport  Port=7
  In8 : Inport  Port=8
  In9 : Inport  Port=9
  In10 : Inport  Port=10
  In11 : Inport  Port=11
  In12 : Inport  Port=12
  Bus Creator : BusCreator  Inputs=22
  Demux{1..10} (10 alike) : Demux  Outputs=2
  Scope : Scope  NumInputPorts=4
  m : Outport
  wires:
  Demux4/2 -> Bus Creator/12  "Psw_Diode2"
  Demux2/2 -> Bus Creator/6  "Psw_IGBT2"
  Demux8/1 -> Bus Creator/20  "Tj_Diode1"
  In2/1 -> Demux9/1
  Demux9/2 -> Bus Creator/4  "V_Dev2"
  In1/1 -> Demux10/1
  Demux1/1 -> Bus Creator/7  "Pcond_IGBT1"
  Demux5/1 -> Bus Creator/13  "Pcond_Diode1"
  Demux2/1 -> Bus Creator/5  "Psw_IGBT1"
  Demux7/2 -> Bus Creator/19  "Tj_IGBT2"
  In11/1 -> Demux8/1
  Demux9/1 -> Bus Creator/3  "I_Dev2"
  In4/1 -> Demux1/1
  In7/1 -> Demux5/1
  Demux10/1 -> Bus Creator/1  "I_Dev1"
  In3/1 -> Demux2/1
  Demux7/1 -> Bus Creator/18  "Tj_IGBT1"
  In9/1 -> Bus Creator/17  "Ptot_HalfBridge"
  In10/1 -> Demux7/1
  Demux4/1 -> Bus Creator/11  "Psw_Diode1"
  In12/1 -> Bus Creator/22  "Tcase"
  Demux6/1 -> Scope/2, [D1], Bus Creator/15  "Ptot_Diode1"
  In8/1 -> Demux6/1
  Demux6/2 -> Scope/1, [D2], Bus Creator/16  "Ptot_Diode2"
  Demux3/2 -> Scope/3, [IGBT2], Bus Creator/10  "Ptot_IGBT2"
  Demux10/2 -> Bus Creator/2  "V_Dev1"
  Demux1/2 -> Bus Creator/8  "Pcond_IGBT2"
  In5/1 -> Demux3/1
  Demux3/1 -> Scope/4, [IGBT1], Bus Creator/9  "Ptot_IGBT1"
  Demux5/2 -> Bus Creator/14  "Pcond_Diode2"
  Bus Creator/1 -> m/1
  Demux8/2 -> Bus Creator/21  "Tj_Diode2"
  In6/1 -> Demux4/1

== system transfer_function_calculation/Generator/3 Level Converter2/Loss Calculation/Leg B1/Subsystem/Loss Calculation Unit ==
  QD1 : Inport
  QD2 : Inport  Port=2
  Add1 : Sum
  Add2 : Sum  Inputs=+
  Add3 : Sum  Inputs=+-
  Add4 : Sum  Inputs=+
  Demux IGBTs and Diodes Currents and voltages : Subsystem
  Diodes Losses Calculation : Subsystem
  Heat Flow Source : fl_lib/Thermal/Thermal Sources/Ideal Heat Flow Source
  IGBTs Losses Calculation : Subsystem
  K1 : Constant  Value=273
  PS-Simulink Converter : nesl_utility/PS-Simulink Converter  PhysicalDomain=network_engine_domain  SubClassName=ps_output  LeftPortType=input  RightPortType=output  PseudoPeriodic=off  Frequencies=[]  Unit=1  AffineConversion=off
  Rate Transition : RateTransition  OutPortSampleTime=Ts_Simscape
  Rate Transition1 : RateTransition  OutPortSampleTime=Ts
  Simulink-PS Converter1 : nesl_utility/Simulink-PS Converter  PhysicalDomain=network_engine_domain  SubClassName=ps_input  LeftPortType=input  RightPortType=output  PseudoPeriodic=off  Frequencies=[]  NoiseDistribution=none  NoiseParameters=[]  Unit=1  AffineConversion=off  InputFiltering=off  SimscapeFilterOrder=1  InputFilterTimeConstant=1e-4  UdotUserProvided=0
  Temperature Sensor : fl_lib/Thermal/Thermal Sensors/Ideal Temperature Sensor
  Thermal Reference1 : fl_lib/Thermal/Thermal Elements/Thermal Reference
  Thermal Reference4 : fl_lib/Thermal/Thermal Elements/Thermal Reference
  Thermal Model : Subsystem  mask(State-Space Thermal Model (Junction-to-Case)){Zth_IGBT=[ IGBT_Rth_jc    IGBT_Cth_j ], Zth_Diode=[ DIODE_Rth_jc    DIODE_Cth_j], Tj0=Tj0, Ts=Ts}
      mask prompts: Zth_IGBT "IGBT Thermal Impedance [ Rth (K/W)  Cth (J/K) ]:"; Zth_Diode "Diode Thermal Impedance [ Rth (K/W)  Cth (J/K) ]:"; Tj0 "Junction Initial Temperature (C)"; Ts "Sample time (s):"
      mask init: same as transfer_function_calculation/Generator/3 Level Converter2/Loss Calculation/Leg A1/Subsystem/Loss Calculation Unit/Thermal Model
  HA1 : PMIOPort  Port=1  Side=Right
  mQd1 : Outport
  mQd2 : Outport  Port=2
  Psw_IGBTs : Outport  Port=3
  Pcond_IGBT : Outport  Port=4
  Ptot_IGBTs : Outport  Port=5
  Psw_Diodes : Outport  Port=6
  Pcond_diodes : Outport  Port=7
  Ptot_Diodes : Outport  Port=8
  Ptot_HB : Outport  Port=9
  TJ_IGBT : Outport  Port=10
  TJ_Diodes : Outport  Port=11
  Tcase : Outport  Port=12
  wires:
  Rate Transition/1 -> Simulink-PS Converter1/1
  Thermal Model/2(Pout) -> Rate Transition/1
  K1/1 -> Add3/2
  PS-Simulink Converter/1 -> Add3/1
  Add3/1 -> Rate Transition1/1, Tcase/1
  Thermal Model/1(Tj_IGBTs) -> IGBTs Losses Calculation/1(Tj_C), TJ_IGBT/1
  Thermal Model/3(Tj_Diodes) -> Diodes Losses Calculation/2(Tj_C), TJ_Diodes/1
  IGBTs Losses Calculation/1(Psw) -> Psw_IGBTs/1
  Diodes Losses Calculation/2(Psw) -> Psw_Diodes/1
  Diodes Losses Calculation/3(Pcond) -> Pcond_diodes/1
  Add1/1 -> Ptot_HB/1
  Add4/1 -> Add1/1
  Add2/1 -> Add1/2
  Rate Transition1/1 -> Thermal Model/3(Tcase)
  Demux IGBTs and Diodes Currents and voltages/2(Diodes) -> Diodes Losses Calculation/1(i,v)
  Demux IGBTs and Diodes Currents and voltages/1(IGBTs) -> IGBTs Losses Calculation/2(i,v)
  QD2/1 -> Demux IGBTs and Diodes Currents and voltages/2(QD2), mQd2/1
  QD1/1 -> Demux IGBTs and Diodes Currents and voltages/1(QD1), mQd1/1
  IGBTs Losses Calculation/2(Pcond) -> Pcond_IGBT/1
  Diodes Losses Calculation/1(Ptot) -> Add2/1, Thermal Model/2(P_Diodes), Ptot_Diodes/1
  IGBTs Losses Calculation/3(Ptot) -> Add4/1, Thermal Model/1(P_IGBTs), Ptot_IGBTs/1
  connections:
  Temperature Sensor/RConn1 -- Thermal Reference1/LConn1
  Temperature Sensor/RConn2 -- PS-Simulink Converter/LConn1
  Simulink-PS Converter1/RConn1 -- Heat Flow Source/RConn1
  Thermal Reference4/LConn1 -- Heat Flow Source/RConn2
  Temperature Sensor/LConn1 -- HA1/RConn1 -- Heat Flow Source/LConn1

== system transfer_function_calculation/Generator/3 Level Converter2/Loss Calculation/Leg B2/Heat Sink (Simscape thermal model)/PS2S ==
  Add1 : Sum  Inputs=+-
  K1 : Constant  Value=273
  PS-Simulink Converter : nesl_utility/PS-Simulink Converter  PhysicalDomain=network_engine_domain  SubClassName=ps_output  LeftPortType=input  RightPortType=output  PseudoPeriodic=off  Frequencies=[]  Unit=1  AffineConversion=off
  In : PMIOPort  Port=1  Side=Left
  Out : Outport
  wires:
  Add1/1 -> Out/1
  PS-Simulink Converter/1 -> Add1/1
  K1/1 -> Add1/2
  connections:
  In/RConn1 -- PS-Simulink Converter/LConn1

== system transfer_function_calculation/Generator/3 Level Converter2/Loss Calculation/Leg B2/Heat Sink (Simscape thermal model)/PS2S1 ==
  Add1 : Sum  Inputs=+-
  K1 : Constant  Value=273
  PS-Simulink Converter : nesl_utility/PS-Simulink Converter  PhysicalDomain=network_engine_domain  SubClassName=ps_output  LeftPortType=input  RightPortType=output  PseudoPeriodic=off  Frequencies=[]  Unit=1  AffineConversion=off
  In : PMIOPort  Port=1  Side=Left
  Out : Outport
  wires:
  K1/1 -> Add1/2
  PS-Simulink Converter/1 -> Add1/1
  Add1/1 -> Out/1
  connections:
  In/RConn1 -- PS-Simulink Converter/LConn1

== system transfer_function_calculation/Generator/3 Level Converter2/Loss Calculation/Leg B2/Heat Sink (Simscape thermal model)/S2PS1 ==
  In : Inport
  Add : Sum
  K2 : Constant  Value=273
  Simulink-PS Converter : nesl_utility/Simulink-PS Converter  PhysicalDomain=network_engine_domain  SubClassName=ps_input  LeftPortType=input  RightPortType=output  PseudoPeriodic=off  Frequencies=[]  NoiseDistribution=none  NoiseParameters=[]  Unit=1  AffineConversion=off  InputFiltering=off  SimscapeFilterOrder=1  InputFilterTimeConstant=1e-4  UdotUserProvided=0
  Out : PMIOPort  Port=1  Side=Right
  wires:
  In/1 -> Add/2
  K2/1 -> Add/1
  Add/1 -> Simulink-PS Converter/1
  connections:
  Out/RConn1 -- Simulink-PS Converter/RConn1

== system transfer_function_calculation/Generator/3 Level Converter2/Loss Calculation/Leg B2/Subsystem/Bus Creator ==
  In1 : Inport
  In2 : Inport  Port=2
  In3 : Inport  Port=3
  In4 : Inport  Port=4
  In5 : Inport  Port=5
  In6 : Inport  Port=6
  In7 : Inport  Port=7
  In8 : Inport  Port=8
  In9 : Inport  Port=9
  In10 : Inport  Port=10
  In11 : Inport  Port=11
  In12 : Inport  Port=12
  Bus Creator : BusCreator  Inputs=22
  Demux{1..10} (10 alike) : Demux  Outputs=2
  Scope : Scope  NumInputPorts=4
  m : Outport
  wires:
  In6/1 -> Demux4/1
  Demux8/2 -> Bus Creator/21  "Tj_Diode2"
  Bus Creator/1 -> m/1
  Demux5/2 -> Bus Creator/14  "Pcond_Diode2"
  Demux3/1 -> Bus Creator/9, [IGBT1], Scope/4  "Ptot_IGBT1"
  In5/1 -> Demux3/1
  Demux1/2 -> Bus Creator/8  "Pcond_IGBT2"
  Demux10/2 -> Bus Creator/2  "V_Dev1"
  Demux3/2 -> Bus Creator/10, [IGBT2], Scope/3  "Ptot_IGBT2"
  Demux6/2 -> Bus Creator/16, [D2], Scope/1  "Ptot_Diode2"
  In8/1 -> Demux6/1
  Demux6/1 -> Bus Creator/15, [D1], Scope/2  "Ptot_Diode1"
  In12/1 -> Bus Creator/22  "Tcase"
  Demux4/1 -> Bus Creator/11  "Psw_Diode1"
  In10/1 -> Demux7/1
  In9/1 -> Bus Creator/17  "Ptot_HalfBridge"
  Demux7/1 -> Bus Creator/18  "Tj_IGBT1"
  In3/1 -> Demux2/1
  Demux10/1 -> Bus Creator/1  "I_Dev1"
  In7/1 -> Demux5/1
  In4/1 -> Demux1/1
  Demux9/1 -> Bus Creator/3  "I_Dev2"
  In11/1 -> Demux8/1
  Demux7/2 -> Bus Creator/19  "Tj_IGBT2"
  Demux2/1 -> Bus Creator/5  "Psw_IGBT1"
  Demux5/1 -> Bus Creator/13  "Pcond_Diode1"
  Demux1/1 -> Bus Creator/7  "Pcond_IGBT1"
  In1/1 -> Demux10/1
  Demux9/2 -> Bus Creator/4  "V_Dev2"
  In2/1 -> Demux9/1
  Demux8/1 -> Bus Creator/20  "Tj_Diode1"
  Demux2/2 -> Bus Creator/6  "Psw_IGBT2"
  Demux4/2 -> Bus Creator/12  "Psw_Diode2"

== system transfer_function_calculation/Generator/3 Level Converter2/Loss Calculation/Leg B2/Subsystem/Loss Calculation Unit ==
  QD1 : Inport
  QD2 : Inport  Port=2
  Add1 : Sum
  Add2 : Sum  Inputs=+
  Add3 : Sum  Inputs=+-
  Add4 : Sum  Inputs=+
  Demux IGBTs and Diodes Currents and voltages : Subsystem
  Diodes Losses Calculation : Subsystem
  Heat Flow Source : fl_lib/Thermal/Thermal Sources/Ideal Heat Flow Source
  IGBTs Losses Calculation : Subsystem
  K1 : Constant  Value=273
  PS-Simulink Converter : nesl_utility/PS-Simulink Converter  PhysicalDomain=network_engine_domain  SubClassName=ps_output  LeftPortType=input  RightPortType=output  PseudoPeriodic=off  Frequencies=[]  Unit=1  AffineConversion=off
  Rate Transition : RateTransition  OutPortSampleTime=Ts_Simscape
  Rate Transition1 : RateTransition  OutPortSampleTime=Ts
  Simulink-PS Converter1 : nesl_utility/Simulink-PS Converter  PhysicalDomain=network_engine_domain  SubClassName=ps_input  LeftPortType=input  RightPortType=output  PseudoPeriodic=off  Frequencies=[]  NoiseDistribution=none  NoiseParameters=[]  Unit=1  AffineConversion=off  InputFiltering=off  SimscapeFilterOrder=1  InputFilterTimeConstant=1e-4  UdotUserProvided=0
  Temperature Sensor : fl_lib/Thermal/Thermal Sensors/Ideal Temperature Sensor
  Thermal Reference1 : fl_lib/Thermal/Thermal Elements/Thermal Reference
  Thermal Reference4 : fl_lib/Thermal/Thermal Elements/Thermal Reference
  Thermal Model : Subsystem  mask(State-Space Thermal Model (Junction-to-Case)){Zth_IGBT=[ IGBT_Rth_jc    IGBT_Cth_j ], Zth_Diode=[ DIODE_Rth_jc    DIODE_Cth_j], Tj0=Tj0, Ts=Ts}
      mask prompts: Zth_IGBT "IGBT Thermal Impedance [ Rth (K/W)  Cth (J/K) ]:"; Zth_Diode "Diode Thermal Impedance [ Rth (K/W)  Cth (J/K) ]:"; Tj0 "Junction Initial Temperature (C)"; Ts "Sample time (s):"
      mask init: same as transfer_function_calculation/Generator/3 Level Converter2/Loss Calculation/Leg A1/Subsystem/Loss Calculation Unit/Thermal Model
  HA1 : PMIOPort  Port=1  Side=Right
  mQd1 : Outport
  mQd2 : Outport  Port=2
  Psw_IGBTs : Outport  Port=3
  Pcond_IGBT : Outport  Port=4
  Ptot_IGBTs : Outport  Port=5
  Psw_Diodes : Outport  Port=6
  Pcond_diodes : Outport  Port=7
  Ptot_Diodes : Outport  Port=8
  Ptot_HB : Outport  Port=9
  TJ_IGBT : Outport  Port=10
  TJ_Diodes : Outport  Port=11
  Tcase : Outport  Port=12
  wires:
  IGBTs Losses Calculation/3(Ptot) -> Ptot_IGBTs/1, Thermal Model/1(P_IGBTs), Add4/1
  Diodes Losses Calculation/1(Ptot) -> Ptot_Diodes/1, Thermal Model/2(P_Diodes), Add2/1
  IGBTs Losses Calculation/2(Pcond) -> Pcond_IGBT/1
  QD1/1 -> mQd1/1, Demux IGBTs and Diodes Currents and voltages/1(QD1)
  QD2/1 -> mQd2/1, Demux IGBTs and Diodes Currents and voltages/2(QD2)
  Demux IGBTs and Diodes Currents and voltages/1(IGBTs) -> IGBTs Losses Calculation/2(i,v)
  Demux IGBTs and Diodes Currents and voltages/2(Diodes) -> Diodes Losses Calculation/1(i,v)
  Rate Transition1/1 -> Thermal Model/3(Tcase)
  Add2/1 -> Add1/2
  Add4/1 -> Add1/1
  Add1/1 -> Ptot_HB/1
  Diodes Losses Calculation/3(Pcond) -> Pcond_diodes/1
  Diodes Losses Calculation/2(Psw) -> Psw_Diodes/1
  IGBTs Losses Calculation/1(Psw) -> Psw_IGBTs/1
  Thermal Model/3(Tj_Diodes) -> TJ_Diodes/1, Diodes Losses Calculation/2(Tj_C)
  Thermal Model/1(Tj_IGBTs) -> TJ_IGBT/1, IGBTs Losses Calculation/1(Tj_C)
  Add3/1 -> Tcase/1, Rate Transition1/1
  PS-Simulink Converter/1 -> Add3/1
  K1/1 -> Add3/2
  Thermal Model/2(Pout) -> Rate Transition/1
  Rate Transition/1 -> Simulink-PS Converter1/1
  connections:
  Heat Flow Source/LConn1 -- HA1/RConn1 -- Temperature Sensor/LConn1
  Thermal Reference4/LConn1 -- Heat Flow Source/RConn2
  Simulink-PS Converter1/RConn1 -- Heat Flow Source/RConn1
  Temperature Sensor/RConn2 -- PS-Simulink Converter/LConn1
  Temperature Sensor/RConn1 -- Thermal Reference1/LConn1

== system transfer_function_calculation/Generator/3 Level Converter2/Loss Calculation/Leg C1/Heat Sink (Simscape thermal model)/PS2S ==
  Add1 : Sum  Inputs=+-
  K1 : Constant  Value=273
  PS-Simulink Converter : nesl_utility/PS-Simulink Converter  PhysicalDomain=network_engine_domain  SubClassName=ps_output  LeftPortType=input  RightPortType=output  PseudoPeriodic=off  Frequencies=[]  Unit=1  AffineConversion=off
  In : PMIOPort  Port=1  Side=Left
  Out : Outport
  wires:
  K1/1 -> Add1/2
  PS-Simulink Converter/1 -> Add1/1
  Add1/1 -> Out/1
  connections:
  In/RConn1 -- PS-Simulink Converter/LConn1

== system transfer_function_calculation/Generator/3 Level Converter2/Loss Calculation/Leg C1/Heat Sink (Simscape thermal model)/PS2S1 ==
  Add1 : Sum  Inputs=+-
  K1 : Constant  Value=273
  PS-Simulink Converter : nesl_utility/PS-Simulink Converter  PhysicalDomain=network_engine_domain  SubClassName=ps_output  LeftPortType=input  RightPortType=output  PseudoPeriodic=off  Frequencies=[]  Unit=1  AffineConversion=off
  In : PMIOPort  Port=1  Side=Left
  Out : Outport
  wires:
  Add1/1 -> Out/1
  PS-Simulink Converter/1 -> Add1/1
  K1/1 -> Add1/2
  connections:
  In/RConn1 -- PS-Simulink Converter/LConn1

== system transfer_function_calculation/Generator/3 Level Converter2/Loss Calculation/Leg C1/Heat Sink (Simscape thermal model)/S2PS1 ==
  In : Inport
  Add : Sum
  K2 : Constant  Value=273
  Simulink-PS Converter : nesl_utility/Simulink-PS Converter  PhysicalDomain=network_engine_domain  SubClassName=ps_input  LeftPortType=input  RightPortType=output  PseudoPeriodic=off  Frequencies=[]  NoiseDistribution=none  NoiseParameters=[]  Unit=1  AffineConversion=off  InputFiltering=off  SimscapeFilterOrder=1  InputFilterTimeConstant=1e-4  UdotUserProvided=0
  Out : PMIOPort  Port=1  Side=Right
  wires:
  Add/1 -> Simulink-PS Converter/1
  K2/1 -> Add/1
  In/1 -> Add/2
  connections:
  Out/RConn1 -- Simulink-PS Converter/RConn1
